simulink subsystem "F16_Quaternion"  (R2023b)
settings: Solver=VariableStepAuto  StartTime=0.0  StopTime=10.0  RelTol=1e-3
undefined symbols (not defined in the file): controlDeflections, dataBase, deltaLEF, e0_0, e1_0, e2_0, e3_0, pm_0, statesFinal, Vm_0, xme_0
libraries: sharedtransform x4, aerolibtransform2 x2, matrix_library x2, shared6dof x1
(part 2 of 2)

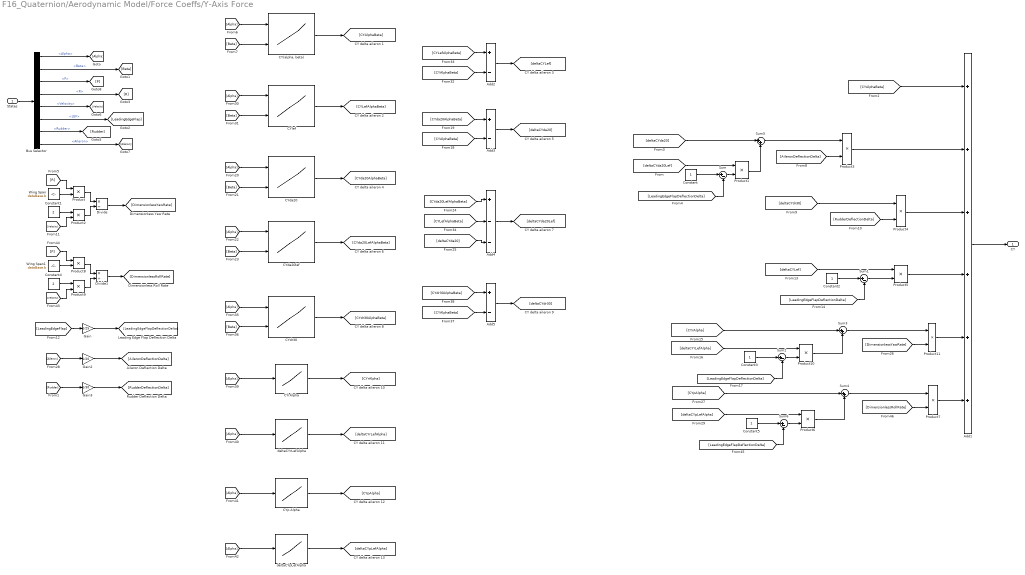
== system F16_Quaternion/Aerodynamic Model/Force Coeffs/Y-Axis Force ==
  States : Inport
  Add1 : Sum  Inputs=++++++
  Add2 : Sum  Inputs=+-
  Add3 : Sum  Inputs=+-
  Add4 : Sum  Inputs=+--
  Add5 : Sum  Inputs=+-
  Bus Selector : BusSelector  OutputSignals=Alpha,Beta,P,R,Velocity,LEF,Rudder,Aileron
  "CY(alpha, beta)" : Lookup_n-D  BreakpointsForDimension1=dataBase.f16_AerodynamicData.BP.CY.CY.alpha  BreakpointsForDimension2=dataBase.f16_AerodynamicData.BP.CY.CY.beta  Table=dataBase.f16_AerodynamicData.data.CY.CY  InternalRulePriority=Speed  RndMeth=Simplest
      settings: InputPortMap=u0,u1
  CYda20 : Lookup_n-D  BreakpointsForDimension1=dataBase.f16_AerodynamicData.BP.CY.CYda20.alpha  BreakpointsForDimension2=dataBase.f16_AerodynamicData.BP.CY.CYda20.beta  Table=dataBase.f16_AerodynamicData.data.CY.CYda20  InternalRulePriority=Speed  RndMeth=Simplest
      settings: InputPortMap=u0,u1
  CYda20lef : Lookup_n-D  BreakpointsForDimension1=dataBase.f16_AerodynamicData.BP.CY.CYda20lef.alpha  BreakpointsForDimension2=dataBase.f16_AerodynamicData.BP.CY.CYda20lef.beta  Table=dataBase.f16_AerodynamicData.data.CY.CYda20lef  InternalRulePriority=Speed  RndMeth=Simplest
      settings: InputPortMap=u0,u1
  CYdr30 : Lookup_n-D  BreakpointsForDimension1=dataBase.f16_AerodynamicData.BP.CY.CYdr30.alpha  BreakpointsForDimension2=dataBase.f16_AerodynamicData.BP.CY.CYdr30.beta  Table=dataBase.f16_AerodynamicData.data.CY.CYdr30  InternalRulePriority=Speed  RndMeth=Simplest
      settings: InputPortMap=u0,u1
  CYlef : Lookup_n-D  BreakpointsForDimension1=dataBase.f16_AerodynamicData.BP.CY.CYlef.alpha  BreakpointsForDimension2=dataBase.f16_AerodynamicData.BP.CY.CYlef.beta  Table=dataBase.f16_AerodynamicData.data.CY.CYlef  InternalRulePriority=Speed  RndMeth=Simplest
      settings: InputPortMap=u0,u1
  CYp Alpha : Lookup_n-D  NumberOfTableDimensions=1  BreakpointsForDimension1=dataBase.f16_AerodynamicData.BP.CY.CYp.alpha  Table=dataBase.f16_AerodynamicData.data.CY.CYp  InternalRulePriority=Speed  RndMeth=Simplest
  CYrAlpha : Lookup_n-D  NumberOfTableDimensions=1  BreakpointsForDimension1=dataBase.f16_AerodynamicData.BP.CY.CYr.alpha  Table=dataBase.f16_AerodynamicData.data.CY.CYr  InternalRulePriority=Speed  RndMeth=Simplest
  Constant{,2..3,5} (4 alike) : Constant
  Constant1 : Constant  Value=2
  Constant4 : Constant  Value=2
  Divide : Product  Inputs=*/
  Divide1 : Product  Inputs=*/
  Gain : Gain  Gain=1/25
  Gain2 : Gain  Gain=1/20
  Gain3 : Gain  Gain=1/30
  Product{,1..11} (12 alike) : Product
  Sum{,1..2,6} (4 alike) : Sum  Inputs=|+-
  Sum3 : Sum  Inputs=|++
  Sum4 : Sum  Inputs=|++
  Sum5 : Sum  Inputs=|++
  Wing Span : Constant  Value=dataBase.b
  Wing Span1 : Constant  Value=dataBase.b
  deltaCYpLefAlpha : Lookup_n-D  NumberOfTableDimensions=1  BreakpointsForDimension1=dataBase.f16_AerodynamicData.BP.CY.deltaCYplef.alpha  Table=dataBase.f16_AerodynamicData.data.CY.deltaCYplef  InternalRulePriority=Speed  RndMeth=Simplest
  deltaCYrLefAlpha : Lookup_n-D  NumberOfTableDimensions=1  BreakpointsForDimension1=dataBase.f16_AerodynamicData.BP.CY.deltaCYrlef.alpha  Table=dataBase.f16_AerodynamicData.data.CY.deltaCYrlef  InternalRulePriority=Speed  RndMeth=Simplest
  CY : Outport  VectorParamsAs1DForOutWhenUnconnected=off
  wires:
  Wing Span/1 -> Product/2
  Divide/1 -> [DimensionlessYawRate]
  [LeadingEdgeFlap] -> Gain/1
  Constant1/1 -> Product2/1
  [Beta] -> "CY(alpha, beta)"/2
  [R] -> Product/1
  States/1 -> Bus Selector/1
  Product2/1 -> Divide/2
  Product/1 -> Divide/1
  [Alpha] -> "CY(alpha, beta)"/1
  Gain/1 -> [LeadingEdgeFlapDeflectionDelta]
  [Velocity] -> Product2/2
  Add1/1 -> CY/1
  "CY(alpha, beta)"/1 -> [CYAlphaBeta]
  [Beta] -> CYda20/2
  [Alpha] -> CYda20/1
  [Alpha] -> CYda20lef/1
  [Beta] -> CYda20lef/2
  [Aileron] -> Gain2/1
  Gain2/1 -> [AileronDeflectionDelta]
  [Alpha] -> CYlef/1
  [Beta] -> CYlef/2
  CYlef/1 -> [CYLefAlphaBeta]
  Add2/1 -> [deltaCYLef]
  [CYAlphaBeta] -> Add2/2
  [CYLefAlphaBeta] -> Add2/1
  CYda20/1 -> [CYda20AlphaBeta]
  [CYda20AlphaBeta] -> Add3/1
  [CYAlphaBeta] -> Add3/2
  Add3/1 -> [deltaCYda20]
  CYda20lef/1 -> [CYda20LefAlphaBeta]
  [CYda20LefAlphaBeta] -> Add4/1
  [CYLefAlphaBeta] -> Add4/2
  [deltaCYda20] -> Add4/3
  Add4/1 -> [deltaCYda20Lef]
  CYdr30/1 -> [CYdr30AlphaBeta]
  [Alpha] -> CYdr30/1
  [Beta] -> CYdr30/2
  Add5/1 -> [deltaCYdr30]
  [CYAlphaBeta] -> Add5/2
  [CYdr30AlphaBeta] -> Add5/1
  [Alpha] -> CYrAlpha/1
  CYrAlpha/1 -> [CYrAlpha]
  deltaCYrLefAlpha/1 -> [deltaCYrLefAlpha]
  [Alpha] -> deltaCYrLefAlpha/1
  [Alpha] -> deltaCYpLefAlpha/1
  deltaCYpLefAlpha/1 -> [deltaCYpLefAlpha]
  CYp Alpha/1 -> [CYpAlpha]
  [Alpha] -> CYp Alpha/1
  [Velocity] -> Product9/2
  Product8/1 -> Divide1/1
  Product9/1 -> Divide1/2
  [P] -> Product8/1
  Constant4/1 -> Product9/1
  Divide1/1 -> [DimensionlessRollRate]
  Wing Span1/1 -> Product8/2
  Gain3/1 -> [RudderDeflectionDelta]
  [Rudder] -> Gain3/1
  [CYAlphaBeta] -> Add1/1
  [deltaCYda20Lef] -> Product1/1
  [deltaCYda20] -> Sum5/1
  Product1/1 -> Sum5/2
  Sum5/1 -> Product3/1
  [AileronDeflectionDelta] -> Product3/2
  Product3/1 -> Add1/2
  [RudderDeflectionDelta] -> Product4/2
  [deltaCYdr30] -> Product4/1
  Product4/1 -> Add1/3
  [deltaCYLef] -> Product5/1
  Product5/1 -> Add1/4
  [CYrAlpha] -> Sum3/1
  [deltaCYrLefAlpha] -> Product10/1
  Product10/1 -> Sum3/2
  [DimensionlessYawRate] -> Product11/2
  Sum3/1 -> Product11/1
  Product11/1 -> Add1/5
  Product7/1 -> Add1/6
  Sum4/1 -> Product7/1
  [DimensionlessRollRate] -> Product7/2
  Product6/1 -> Sum4/2
  [deltaCYpLefAlpha] -> Product6/1
  [CYpAlpha] -> Sum4/1
  Constant/1 -> Sum/1
  [LeadingEdgeFlapDeflectionDelta] -> Sum/2
  Sum/1 -> Product1/2
  Constant2/1 -> Sum1/1
  [LeadingEdgeFlapDeflectionDelta] -> Sum1/2
  Sum1/1 -> Product5/2
  Constant3/1 -> Sum2/1
  [LeadingEdgeFlapDeflectionDelta] -> Sum2/2
  Sum2/1 -> Product10/2
  Constant5/1 -> Sum6/1
  [LeadingEdgeFlapDeflectionDelta] -> Sum6/2
  Sum6/1 -> Product6/2
  Bus Selector/1 -> [Alpha]  "<Alpha>"
  Bus Selector/2 -> [Beta]  "<Beta>"
  Bus Selector/3 -> [P]  "<P>"
  Bus Selector/4 -> [R]  "<R>"
  Bus Selector/5 -> [Velocity]  "<Velocity>"
  Bus Selector/6 -> [LeadingEdgeFlap]  "<LEF>"
  Bus Selector/7 -> [Rudder]  "<Rudder>"
  Bus Selector/8 -> [Aileron]  "<Aileron>"

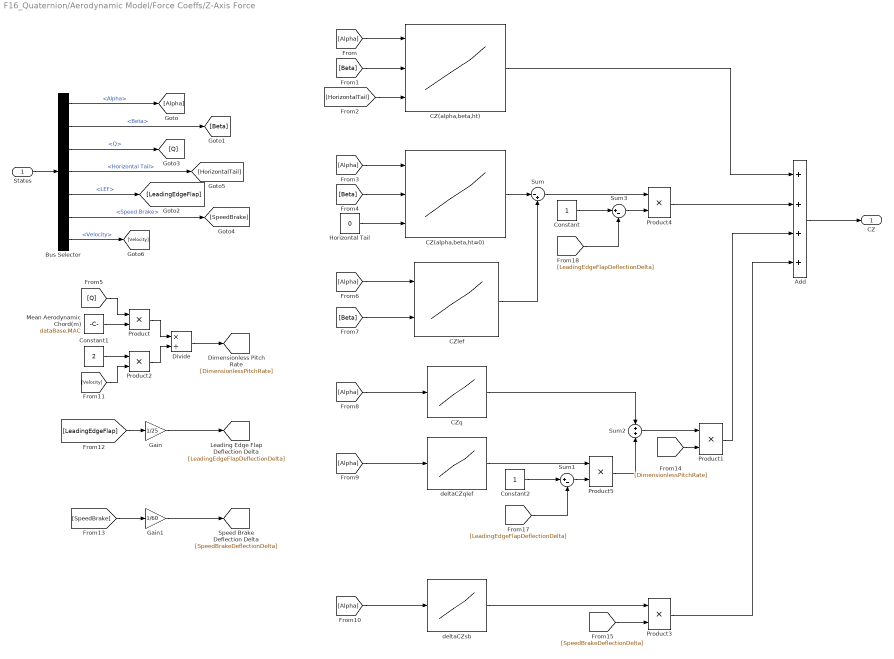
== system F16_Quaternion/Aerodynamic Model/Force Coeffs/Z-Axis Force ==
  States : Inport
  Add : Sum  Inputs=++++
  Bus Selector : BusSelector  OutputSignals=Alpha,Beta,Q,Horizontal Tail,LEF,Speed Brake,Velocity
  CZ(alpha,beta,ht) : Lookup_n-D  NumberOfTableDimensions=3  BreakpointsForDimension1=dataBase.f16_AerodynamicData.BP.CZ.CZ.alpha  BreakpointsForDimension2=dataBase.f16_AerodynamicData.BP.CZ.CZ.beta  BreakpointsForDimension3=dataBase.f16_AerodynamicData.BP.CZ.CZ.dHT  Table=dataBase.f16_AerodynamicData.data.CZ.CZ  InternalRulePriority=Speed  RndMeth=Simplest
      settings: InputPortMap=u0,u1,u2
  CZ(alpha,beta,ht=0) : Lookup_n-D  NumberOfTableDimensions=3  BreakpointsForDimension1=dataBase.f16_AerodynamicData.BP.CZ.CZ.alpha  BreakpointsForDimension2=dataBase.f16_AerodynamicData.BP.CZ.CZ.beta  BreakpointsForDimension3=dataBase.f16_AerodynamicData.BP.CZ.CZ.dHT  Table=dataBase.f16_AerodynamicData.data.CZ.CZ  InternalRulePriority=Speed  RndMeth=Simplest
      settings: InputPortMap=u0,u1,u2
  CZlef : Lookup_n-D  BreakpointsForDimension1=dataBase.f16_AerodynamicData.BP.CZ.CZlef.alpha  BreakpointsForDimension2=dataBase.f16_AerodynamicData.BP.CZ.CZlef.beta  Table=dataBase.f16_AerodynamicData.data.CZ.CZlef  InternalRulePriority=Speed  RndMeth=Simplest
      settings: InputPortMap=u0,u1
  CZq : Lookup_n-D  NumberOfTableDimensions=1  BreakpointsForDimension1=dataBase.f16_AerodynamicData.BP.CZ.CZq.alpha  Table=dataBase.f16_AerodynamicData.data.CZ.CZq  InternalRulePriority=Speed  RndMeth=Simplest
  Constant : Constant
  Constant1 : Constant  Value=2
  Constant2 : Constant
  Divide : Product  Inputs=*/
  Gain : Gain  Gain=1/25
  Gain1 : Gain  Gain=1/60
  Horizontal Tail : Constant  Value=0
  Mean Aerodynamic Chord(m) : Constant  Value=dataBase.MAC
  Product{,1..5} (6 alike) : Product
  Sum : Sum  Inputs=|-+
  Sum1 : Sum  Inputs=|+-
  Sum2 : Sum  Inputs=+|+
  Sum3 : Sum  Inputs=|+-
  deltaCZqlef : Lookup_n-D  NumberOfTableDimensions=1  BreakpointsForDimension1=dataBase.f16_AerodynamicData.BP.CZ.deltaCZqlef.alpha  Table=dataBase.f16_AerodynamicData.data.CZ.deltaCZqlef  InternalRulePriority=Speed  RndMeth=Simplest
  deltaCZsb : Lookup_n-D  NumberOfTableDimensions=1  BreakpointsForDimension1=dataBase.f16_AerodynamicData.BP.CZ.deltaCZSB.alpha  Table=dataBase.f16_AerodynamicData.data.CZ.deltaCZSB  InternalRulePriority=Speed  RndMeth=Simplest
  CZ : Outport  VectorParamsAs1DForOutWhenUnconnected=off
  wires:
  [Beta] -> CZ(alpha,beta,ht=0)/2
  Product2/1 -> Divide/2
  [Alpha] -> CZlef/1
  [Velocity] -> Product2/2
  Sum2/1 -> Product1/1
  [SpeedBrake] -> Gain1/1
  Product/1 -> Divide/1
  [LeadingEdgeFlap] -> Gain/1
  Divide/1 -> [DimensionlessPitchRate]
  Mean Aerodynamic Chord(m)/1 -> Product/2
  [Alpha] -> deltaCZsb/1
  [HorizontalTail] -> CZ(alpha,beta,ht)/3
  CZlef/1 -> Sum/2
  Constant1/1 -> Product2/1
  [Beta] -> CZ(alpha,beta,ht)/2
  Horizontal Tail/1 -> CZ(alpha,beta,ht=0)/3
  [Alpha] -> CZ(alpha,beta,ht=0)/1
  [Alpha] -> CZq/1
  [Alpha] -> deltaCZqlef/1
  [Alpha] -> CZ(alpha,beta,ht)/1
  States/1 -> Bus Selector/1
  CZ(alpha,beta,ht=0)/1 -> Sum/1
  Sum/1 -> Product4/1
  Product3/1 -> Add/4
  CZq/1 -> Sum2/1
  Gain1/1 -> [SpeedBrakeDeflectionDelta]
  CZ(alpha,beta,ht)/1 -> Add/1
  Add/1 -> CZ/1
  deltaCZsb/1 -> Product3/1
  [SpeedBrakeDeflectionDelta] -> Product3/2
  [Q] -> Product/1
  [DimensionlessPitchRate] -> Product1/2
  [Beta] -> CZlef/2
  Product1/1 -> Add/3
  Gain/1 -> [LeadingEdgeFlapDeflectionDelta]
  Product4/1 -> Add/2
  deltaCZqlef/1 -> Product5/1
  Product5/1 -> Sum2/2
  Sum3/1 -> Product4/2
  [LeadingEdgeFlapDeflectionDelta] -> Sum3/2
  Constant/1 -> Sum3/1
  Sum1/1 -> Product5/2
  [LeadingEdgeFlapDeflectionDelta] -> Sum1/2
  Constant2/1 -> Sum1/1
  Bus Selector/1 -> [Alpha]  "<Alpha>"
  Bus Selector/2 -> [Beta]  "<Beta>"
  Bus Selector/3 -> [Q]  "<Q>"
  Bus Selector/4 -> [HorizontalTail]  "<Horizontal Tail>"
  Bus Selector/5 -> [LeadingEdgeFlap]  "<LEF>"
  Bus Selector/7 -> [Velocity]  "<Velocity>"
  Bus Selector/6 -> [SpeedBrake]  "<Speed Brake>"

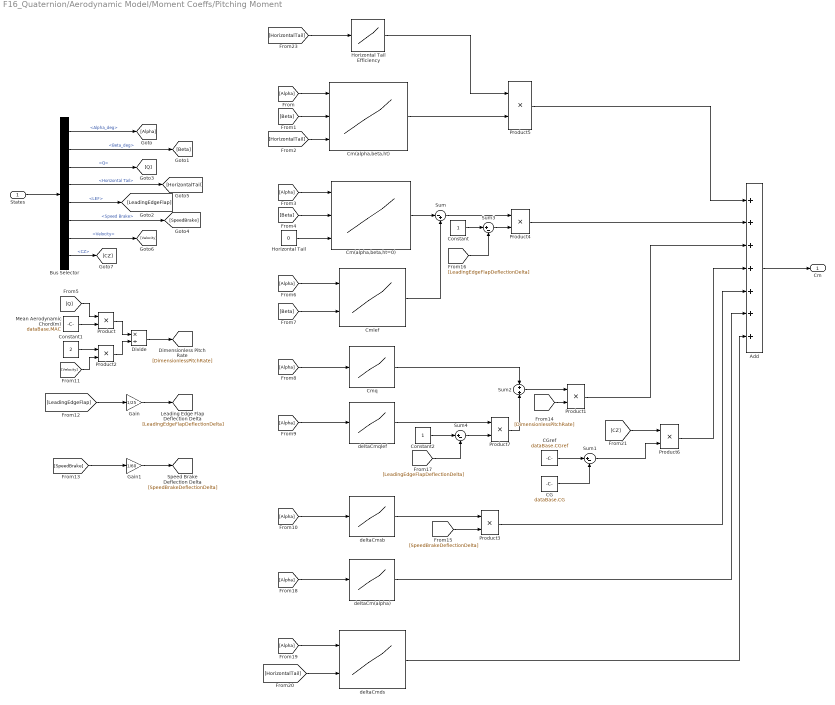
== system F16_Quaternion/Aerodynamic Model/Moment Coeffs/Pitching Moment ==
  States : Inport
  Add : Sum  Inputs=+++++++
  Bus Selector : BusSelector  OutputSignals=Alpha_deg,Beta_deg,Q,Horizontal Tail,LEF,Speed Brake,Velocity,CZ
  CG : Constant  Value=dataBase.CG
  CGref : Constant  Value=dataBase.CGref
  Cm(alpha,beta,ht) : Lookup_n-D  NumberOfTableDimensions=3  BreakpointsForDimension1=dataBase.f16_AerodynamicData.BP.Cm.Cm.alpha  BreakpointsForDimension2=dataBase.f16_AerodynamicData.BP.Cm.Cm.beta  BreakpointsForDimension3=dataBase.f16_AerodynamicData.BP.Cm.Cm.dHT  Table=dataBase.f16_AerodynamicData.data.Cm.Cm  ExtrapMethod=Clip  InternalRulePriority=Speed  RndMeth=Simplest
      settings: InputPortMap=u0,u1,u2
  Cm(alpha,beta,ht=0) : Lookup_n-D  NumberOfTableDimensions=3  BreakpointsForDimension1=dataBase.f16_AerodynamicData.BP.Cm.Cm.alpha  BreakpointsForDimension2=dataBase.f16_AerodynamicData.BP.Cm.Cm.beta  BreakpointsForDimension3=dataBase.f16_AerodynamicData.BP.Cm.Cm.dHT  Table=dataBase.f16_AerodynamicData.data.Cm.Cm  ExtrapMethod=Clip  InternalRulePriority=Speed  RndMeth=Simplest
      settings: InputPortMap=u0,u1,u2
  Cmlef : Lookup_n-D  BreakpointsForDimension1=dataBase.f16_AerodynamicData.BP.Cm.Cmlef.alpha  BreakpointsForDimension2=dataBase.f16_AerodynamicData.BP.Cm.Cmlef.beta  Table=dataBase.f16_AerodynamicData.data.Cm.Cmlef  ExtrapMethod=Clip  InternalRulePriority=Speed  RndMeth=Simplest
      settings: InputPortMap=u0,u1
  Cmq : Lookup_n-D  NumberOfTableDimensions=1  BreakpointsForDimension1=dataBase.f16_AerodynamicData.BP.Cm.Cmq.alpha  Table=dataBase.f16_AerodynamicData.data.Cm.Cmq  ExtrapMethod=Clip  InternalRulePriority=Speed  RndMeth=Simplest
  Constant : Constant
  Constant1 : Constant  Value=2
  Constant2 : Constant
  Divide : Product  Inputs=*/
  Gain : Gain  Gain=1/25
  Gain1 : Gain  Gain=1/60
  Horizontal Tail : Constant  Value=0
  Horizontal Tail Efficiency : Lookup_n-D  NumberOfTableDimensions=1  BreakpointsForDimension1=dataBase.f16_AerodynamicData.BP.Cm.n_dHT.dHT  Table=dataBase.f16_AerodynamicData.data.Cm.n_dHT  ExtrapMethod=Clip  InternalRulePriority=Speed  RndMeth=Simplest
  Mean Aerodynamic Chord(m) : Constant  Value=dataBase.MAC
  Product{,1..7} (8 alike) : Product
  Sum : Sum  Inputs=|-+
  Sum1 : Sum  Inputs=|+-
  Sum2 : Sum  Inputs=+|+
  Sum3 : Sum  Inputs=|+-
  Sum4 : Sum  Inputs=|+-
  deltaCm(alpha) : Lookup_n-D  NumberOfTableDimensions=1  BreakpointsForDimension1=dataBase.f16_AerodynamicData.BP.Cm.deltaCm.alpha  Table=dataBase.f16_AerodynamicData.data.Cm.deltaCm  ExtrapMethod=Clip  InternalRulePriority=Speed  RndMeth=Simplest
  deltaCmds : Lookup_n-D  BreakpointsForDimension1=dataBase.f16_AerodynamicData.BP.Cm.deltaCmds.alpha  BreakpointsForDimension2=dataBase.f16_AerodynamicData.BP.Cm.deltaCmds.dHT  Table=dataBase.f16_AerodynamicData.data.Cm.deltaCmds  ExtrapMethod=Clip  InternalRulePriority=Speed  RndMeth=Simplest
      settings: InputPortMap=u0,u1
  deltaCmqlef : Lookup_n-D  NumberOfTableDimensions=1  BreakpointsForDimension1=dataBase.f16_AerodynamicData.BP.Cm.deltaCmqlef.alpha  Table=dataBase.f16_AerodynamicData.data.Cm.deltaCmqlef  ExtrapMethod=Clip  InternalRulePriority=Speed  RndMeth=Simplest
  deltaCmsb : Lookup_n-D  NumberOfTableDimensions=1  BreakpointsForDimension1=dataBase.f16_AerodynamicData.BP.Cm.deltaCmSB.alpha  Table=dataBase.f16_AerodynamicData.data.Cm.deltaCmSB  ExtrapMethod=Clip  InternalRulePriority=Speed  RndMeth=Simplest
  Cm : Outport
  wires:
  [Beta] -> Cm(alpha,beta,ht=0)/2
  [SpeedBrakeDeflectionDelta] -> Product3/2
  Constant1/1 -> Product2/1
  [Alpha] -> Cm(alpha,beta,ht=0)/1
  Product/1 -> Divide/1
  Cm(alpha,beta,ht=0)/1 -> Sum/1
  Horizontal Tail/1 -> Cm(alpha,beta,ht=0)/3
  [Alpha] -> Cm(alpha,beta,ht)/1
  States/1 -> Bus Selector/1
  [Alpha] -> Cmlef/1
  [Alpha] -> deltaCmqlef/1
  [Alpha] -> Cmq/1
  Mean Aerodynamic Chord(m)/1 -> Product/2
  Product1/1 -> Add/3
  Sum2/1 -> Product1/1
  [Q] -> Product/1
  Gain1/1 -> [SpeedBrakeDeflectionDelta]
  Cmlef/1 -> Sum/2
  [DimensionlessPitchRate] -> Product1/2
  [Beta] -> Cm(alpha,beta,ht)/2
  Divide/1 -> [DimensionlessPitchRate]
  Product4/1 -> Add/2
  Add/1 -> Cm/1
  [LeadingEdgeFlap] -> Gain/1
  [HorizontalTail] -> Cm(alpha,beta,ht)/3
  [SpeedBrake] -> Gain1/1
  Product2/1 -> Divide/2
  Gain/1 -> [LeadingEdgeFlapDeflectionDelta]
  [Velocity] -> Product2/2
  deltaCmsb/1 -> Product3/1
  Sum/1 -> Product4/1
  [Alpha] -> deltaCmsb/1
  Cmq/1 -> Sum2/1
  [Beta] -> Cmlef/2
  [Alpha] -> deltaCm(alpha)/1
  [HorizontalTail] -> deltaCmds/2
  [Alpha] -> deltaCmds/1
  Product5/1 -> Add/1
  [CZ] -> Product6/1
  CGref/1 -> Sum1/1
  CG/1 -> Sum1/2
  deltaCmqlef/1 -> Product7/1
  Product7/1 -> Sum2/2
  [HorizontalTail] -> Horizontal Tail Efficiency/1
  Cm(alpha,beta,ht)/1 -> Product5/2
  Horizontal Tail Efficiency/1 -> Product5/1
  Constant/1 -> Sum3/1
  [LeadingEdgeFlapDeflectionDelta] -> Sum3/2
  Sum3/1 -> Product4/2
  Constant2/1 -> Sum4/1
  Sum4/1 -> Product7/2
  [LeadingEdgeFlapDeflectionDelta] -> Sum4/2
  Product6/1 -> Add/4
  Product3/1 -> Add/5
  deltaCm(alpha)/1 -> Add/6
  deltaCmds/1 -> Add/7
  Bus Selector/1 -> [Alpha]  "<Alpha_deg>"
  Bus Selector/2 -> [Beta]  "<Beta_deg>"
  Bus Selector/3 -> [Q]  "<Q>"
  Bus Selector/4 -> [HorizontalTail]  "<Horizontal Tail>"
  Bus Selector/5 -> [LeadingEdgeFlap]  "<LEF>"
  Bus Selector/6 -> [SpeedBrake]  "<Speed Brake>"
  Bus Selector/7 -> [Velocity]  "<Velocity>"
  Bus Selector/8 -> [CZ]  "<CZ>"
  Sum1/1 -> Product6/2

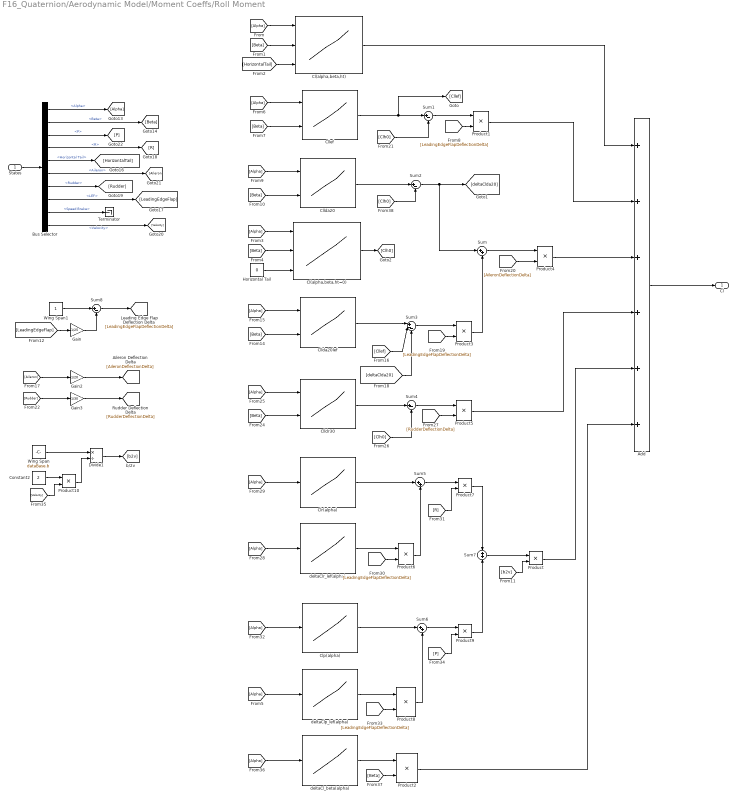
== system F16_Quaternion/Aerodynamic Model/Moment Coeffs/Roll Moment ==
  States : Inport
  Add : Sum  Inputs=++++++
  Bus Selector : BusSelector  OutputSignals=Alpha,Beta,P,R,Horizontal Tail,Aileron,Rudder,LEF,Speed Brake,Velocity
  Cl(alpha,beta,ht) : Lookup_n-D  NumberOfTableDimensions=3  BreakpointsForDimension1=dataBase.f16_AerodynamicData.BP.Cl.Cl.alpha  BreakpointsForDimension2=dataBase.f16_AerodynamicData.BP.Cl.Cl.beta  BreakpointsForDimension3=dataBase.f16_AerodynamicData.BP.Cl.Cl.dHT  Table=dataBase.f16_AerodynamicData.data.Cl.Cl  ExtrapMethod=Clip  InternalRulePriority=Speed  RndMeth=Simplest
      settings: InputPortMap=u0,u1,u2
  Cl(alpha,beta,ht=0) : Lookup_n-D  NumberOfTableDimensions=3  BreakpointsForDimension1=dataBase.f16_AerodynamicData.BP.Cl.Cl.alpha  BreakpointsForDimension2=dataBase.f16_AerodynamicData.BP.Cl.Cl.beta  BreakpointsForDimension3=dataBase.f16_AerodynamicData.BP.Cl.Cl.dHT  Table=dataBase.f16_AerodynamicData.data.Cl.Cl  ExtrapMethod=Clip  InternalRulePriority=Speed  RndMeth=Simplest
      settings: InputPortMap=u0,u1,u2
  Cllda20 : Lookup_n-D  BreakpointsForDimension1=dataBase.f16_AerodynamicData.BP.Cl.Clda20.alpha  BreakpointsForDimension2=dataBase.f16_AerodynamicData.BP.Cl.Clda20.beta  Table=dataBase.f16_AerodynamicData.data.Cl.Clda20  ExtrapMethod=Clip  InternalRulePriority=Speed  RndMeth=Simplest
      settings: InputPortMap=u0,u1
  Cllda20lef : Lookup_n-D  BreakpointsForDimension1=dataBase.f16_AerodynamicData.BP.Cl.Clda20lef.alpha  BreakpointsForDimension2=dataBase.f16_AerodynamicData.BP.Cl.Clda20lef.beta  Table=dataBase.f16_AerodynamicData.data.Cl.Clda20lef  ExtrapMethod=Clip  InternalRulePriority=Speed  RndMeth=Simplest
      settings: InputPortMap=u0,u1
  Clldr30 : Lookup_n-D  BreakpointsForDimension1=dataBase.f16_AerodynamicData.BP.Cl.Cldr30.alpha  BreakpointsForDimension2=dataBase.f16_AerodynamicData.BP.Cl.Cldr30.beta  Table=dataBase.f16_AerodynamicData.data.Cl.Cldr30  ExtrapMethod=Clip  InternalRulePriority=Speed  RndMeth=Simplest
      settings: InputPortMap=u0,u1
  Cllef : Lookup_n-D  BreakpointsForDimension1=dataBase.f16_AerodynamicData.BP.Cl.Cllef.alpha  BreakpointsForDimension2=dataBase.f16_AerodynamicData.BP.Cl.Cllef.beta  Table=dataBase.f16_AerodynamicData.data.Cl.Cllef  ExtrapMethod=Clip  InternalRulePriority=Speed  RndMeth=Simplest
      settings: InputPortMap=u0,u1
  Clp(alpha) : Lookup_n-D  NumberOfTableDimensions=1  BreakpointsForDimension1=dataBase.f16_AerodynamicData.BP.Cl.Clp.alpha  BreakpointsForDimension2=dataBase.f16_AerodynamicData.BP.Cl.Cldr30.beta  Table=dataBase.f16_AerodynamicData.data.Cl.Clp  ExtrapMethod=Clip  InternalRulePriority=Speed  RndMeth=Simplest
  Clr(alpha) : Lookup_n-D  NumberOfTableDimensions=1  BreakpointsForDimension1=dataBase.f16_AerodynamicData.BP.Cl.Clr.alpha  BreakpointsForDimension2=dataBase.f16_AerodynamicData.BP.Cl.Cldr30.beta  Table=dataBase.f16_AerodynamicData.data.Cl.Clr  ExtrapMethod=Clip  InternalRulePriority=Speed  RndMeth=Simplest
  Constant2 : Constant  Value=2
  Divide1 : Product  Inputs=*/
  Gain : Gain  Gain=1/25
  Gain2 : Gain  Gain=1/20
  Gain3 : Gain  Gain=1/30
  Horizontal Tail : Constant  Value=0
  Product{,1..10} (11 alike) : Product
  Sum : Sum  Inputs=|++
  Sum{1..2,4,8} (4 alike) : Sum  Inputs=|+-
  Sum3 : Sum  Inputs=|+--
  Sum5 : Sum  Inputs=|++
  Sum6 : Sum  Inputs=|++
  Sum7 : Sum  Inputs=+|+
  Terminator : Terminator
  Wing Span : Constant  Value=dataBase.b
  Wing Span1 : Constant
  deltaCl_beta(alpha) : Lookup_n-D  NumberOfTableDimensions=1  BreakpointsForDimension1=dataBase.f16_AerodynamicData.BP.Cl.deltaClBeta.alpha  BreakpointsForDimension2=dataBase.f16_AerodynamicData.BP.Cl.Cldr30.beta  Table=dataBase.f16_AerodynamicData.data.Cl.deltaClBeta  ExtrapMethod=Clip  InternalRulePriority=Speed  RndMeth=Simplest
  deltaClp_lef(alpha) : Lookup_n-D  NumberOfTableDimensions=1  BreakpointsForDimension1=dataBase.f16_AerodynamicData.BP.Cl.deltaClplef.alpha  BreakpointsForDimension2=dataBase.f16_AerodynamicData.BP.Cl.Cldr30.beta  Table=dataBase.f16_AerodynamicData.data.Cl.deltaClplef  ExtrapMethod=Clip  InternalRulePriority=Speed  RndMeth=Simplest
  deltaClr_lef(alpha) : Lookup_n-D  NumberOfTableDimensions=1  BreakpointsForDimension1=dataBase.f16_AerodynamicData.BP.Cl.deltaClrlef.alpha  BreakpointsForDimension2=dataBase.f16_AerodynamicData.BP.Cl.Cldr30.beta  Table=dataBase.f16_AerodynamicData.data.Cl.deltaClrlef  ExtrapMethod=Clip  InternalRulePriority=Speed  RndMeth=Simplest
  Cl : Outport
  wires:
  [Beta] -> Cllef/2
  [HorizontalTail] -> Cl(alpha,beta,ht)/3
  Cl(alpha,beta,ht)/1 -> Add/1
  [Alpha] -> Cllef/1
  [Alpha] -> Cl(alpha,beta,ht)/1
  [Beta] -> Cl(alpha,beta,ht)/2
  Add/1 -> Cl/1
  Gain/1 -> Sum8/2
  [LeadingEdgeFlap] -> Gain/1
  [Aileron] -> Gain2/1
  Gain2/1 -> [AileronDeflectionDelta]
  Gain3/1 -> [RudderDeflectionDelta]
  [Rudder] -> Gain3/1
  [Beta] -> Cl(alpha,beta,ht=0)/2
  Horizontal Tail/1 -> Cl(alpha,beta,ht=0)/3
  [Alpha] -> Cl(alpha,beta,ht=0)/1
  Cllef/1 -> Sum1/1, [Cllef]
  [LeadingEdgeFlapDeflectionDelta] -> Product1/2
  Sum1/1 -> Product1/1
  Cl(alpha,beta,ht=0)/1 -> [Clh0]
  [Beta] -> Cllda20/2
  [Alpha] -> Cllda20/1
  Cllda20/1 -> Sum2/1
  Product1/1 -> Add/2
  Sum2/1 -> Sum/1, [deltaClda20]
  [Alpha] -> Cllda20lef/1
  [Beta] -> Cllda20lef/2
  Cllda20lef/1 -> Sum3/1
  [Cllef] -> Sum3/2
  [deltaClda20] -> Sum3/3
  [LeadingEdgeFlapDeflectionDelta] -> Product3/2
  Sum3/1 -> Product3/1
  Product3/1 -> Sum/2
  [AileronDeflectionDelta] -> Product4/2
  Sum/1 -> Product4/1
  Product4/1 -> Add/3
  [Clh0] -> Sum1/2
  [Clh0] -> Sum2/2
  [Alpha] -> Clldr30/1
  [Beta] -> Clldr30/2
  Clldr30/1 -> Sum4/1
  [Clh0] -> Sum4/2
  [RudderDeflectionDelta] -> Product5/2
  Sum4/1 -> Product5/1
  Product5/1 -> Add/4
  [Alpha] -> Clr(alpha)/1
  Clr(alpha)/1 -> Sum5/1
  [Alpha] -> deltaClr_lef(alpha)/1
  [LeadingEdgeFlapDeflectionDelta] -> Product6/2
  deltaClr_lef(alpha)/1 -> Product6/1
  Product6/1 -> Sum5/2
  [Alpha] -> Clp(alpha)/1
  [Alpha] -> deltaClp_lef(alpha)/1
  [LeadingEdgeFlapDeflectionDelta] -> Product8/2
  deltaClp_lef(alpha)/1 -> Product8/1
  Product8/1 -> Sum6/2
  Clp(alpha)/1 -> Sum6/1
  Sum6/1 -> Product9/1
  [P] -> Product9/2
  Sum5/1 -> Product7/1
  [R] -> Product7/2
  Product7/1 -> Sum7/1
  Product9/1 -> Sum7/2
  [Velocity] -> Product10/2
  Constant2/1 -> Product10/1
  Product10/1 -> Divide1/2
  Wing Span/1 -> Divide1/1
  Divide1/1 -> [b2v]
  Sum7/1 -> Product/1
  [b2v] -> Product/2
  [Alpha] -> deltaCl_beta(alpha)/1
  deltaCl_beta(alpha)/1 -> Product2/1
  [Beta] -> Product2/2
  Product/1 -> Add/5
  Product2/1 -> Add/6
  Bus Selector/7 -> [Rudder]  "<Rudder>"
  Bus Selector/3 -> [P]  "<P>"
  Bus Selector/5 -> [HorizontalTail]  "<Horizontal Tail>"
  States/1 -> Bus Selector/1
  Bus Selector/2 -> [Beta]  "<Beta>"
  Bus Selector/10 -> [Velocity]  "<Velocity>"
  Bus Selector/1 -> [Alpha]  "<Alpha>"
  Bus Selector/6 -> [Aileron]  "<Aileron>"
  Bus Selector/8 -> [LeadingEdgeFlap]  "<LEF>"
  Bus Selector/4 -> [R]  "<R>"
  Bus Selector/9 -> Terminator/1  "<Speed Brake>"
  Wing Span1/1 -> Sum8/1
  Sum8/1 -> [LeadingEdgeFlapDeflectionDelta]

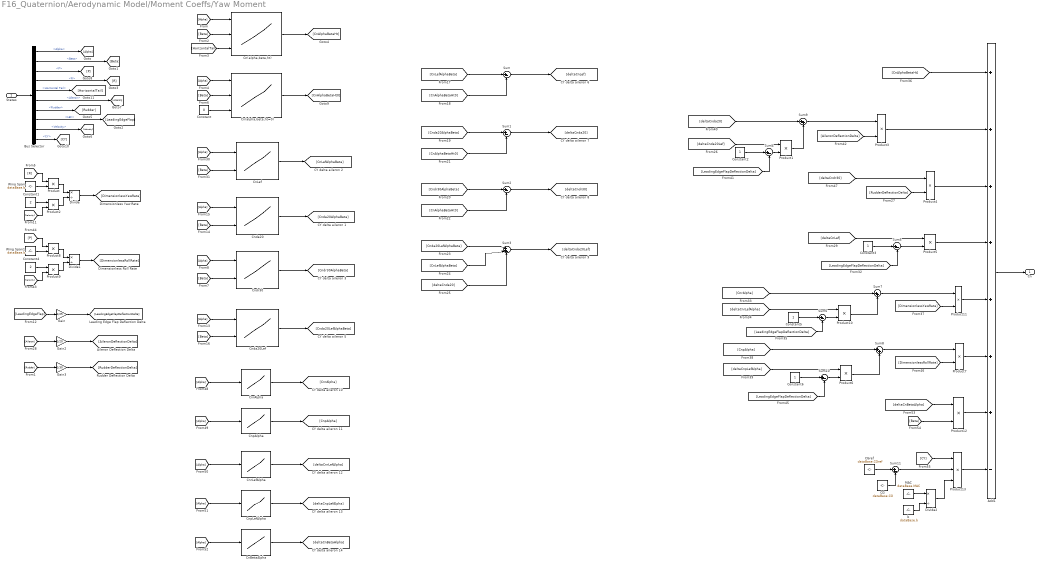
== system F16_Quaternion/Aerodynamic Model/Moment Coeffs/Yaw Moment ==
  States : Inport
  Add1 : Sum  Inputs=+++++++-
  Bus Selector : BusSelector  OutputSignals=Alpha,Beta,P,R,Horizontal Tail,Aileron,Rudder,LEF,Velocity,CY
  CG : Constant  Value=dataBase.CG
  CGref : Constant  Value=dataBase.CGref
  Cn(alpha,beta,ht) : Lookup_n-D  NumberOfTableDimensions=3  BreakpointsForDimension1=dataBase.f16_AerodynamicData.BP.Cn.Cn.alpha  BreakpointsForDimension2=dataBase.f16_AerodynamicData.BP.Cn.Cn.beta  BreakpointsForDimension3=dataBase.f16_AerodynamicData.BP.Cn.Cn.dHT  Table=dataBase.f16_AerodynamicData.data.Cn.Cn  ExtrapMethod=Clip  InternalRulePriority=Speed  RndMeth=Simplest
      settings: InputPortMap=u0,u1,u2
  Cn(alpha,beta,ht=0) : Lookup_n-D  NumberOfTableDimensions=3  BreakpointsForDimension1=dataBase.f16_AerodynamicData.BP.Cn.Cn.alpha  BreakpointsForDimension2=dataBase.f16_AerodynamicData.BP.Cn.Cn.beta  BreakpointsForDimension3=dataBase.f16_AerodynamicData.BP.Cn.Cn.dHT  Table=dataBase.f16_AerodynamicData.data.Cn.Cn  ExtrapMethod=Clip  InternalRulePriority=Speed  RndMeth=Simplest
      settings: InputPortMap=u0,u1,u2
  CnBetaAlpha : Lookup_n-D  NumberOfTableDimensions=1  BreakpointsForDimension1=dataBase.f16_AerodynamicData.BP.Cn.deltaCnBeta.alpha  Table=dataBase.f16_AerodynamicData.data.Cn.deltaCnBeta  ExtrapMethod=Clip  InternalRulePriority=Speed  RndMeth=Simplest
  CnLef : Lookup_n-D  BreakpointsForDimension1=dataBase.f16_AerodynamicData.BP.Cn.Cnlef.alpha  BreakpointsForDimension2=dataBase.f16_AerodynamicData.BP.Cn.Cnlef.beta  Table=dataBase.f16_AerodynamicData.data.Cn.Cnlef  ExtrapMethod=Clip  InternalRulePriority=Speed  RndMeth=Simplest
      settings: InputPortMap=u0,u1
  Cnda20 : Lookup_n-D  BreakpointsForDimension1=dataBase.f16_AerodynamicData.BP.Cn.Cnda20.alpha  BreakpointsForDimension2=dataBase.f16_AerodynamicData.BP.Cn.Cnda20.beta  Table=dataBase.f16_AerodynamicData.data.Cn.Cnda20  ExtrapMethod=Clip  InternalRulePriority=Speed  RndMeth=Simplest
      settings: InputPortMap=u0,u1
  Cnda20Lef : Lookup_n-D  BreakpointsForDimension1=dataBase.f16_AerodynamicData.BP.Cn.Cnda20lef.alpha  BreakpointsForDimension2=dataBase.f16_AerodynamicData.BP.Cn.Cnda20lef.beta  Table=dataBase.f16_AerodynamicData.data.Cn.Cnda20lef  ExtrapMethod=Clip  InternalRulePriority=Speed  RndMeth=Simplest
      settings: InputPortMap=u0,u1
  Cndr30 : Lookup_n-D  BreakpointsForDimension1=dataBase.f16_AerodynamicData.BP.Cn.Cndr30.alpha  BreakpointsForDimension2=dataBase.f16_AerodynamicData.BP.Cn.Cndr30.beta  Table=dataBase.f16_AerodynamicData.data.Cn.Cndr30  ExtrapMethod=Clip  InternalRulePriority=Speed  RndMeth=Simplest
      settings: InputPortMap=u0,u1
  CnpAlpha : Lookup_n-D  NumberOfTableDimensions=1  BreakpointsForDimension1=dataBase.f16_AerodynamicData.BP.Cn.Cnp.alpha  Table=dataBase.f16_AerodynamicData.data.Cn.Cnp  ExtrapMethod=Clip  InternalRulePriority=Speed  RndMeth=Simplest
  CnpLefAlpha : Lookup_n-D  NumberOfTableDimensions=1  BreakpointsForDimension1=dataBase.f16_AerodynamicData.BP.Cn.deltaCnplef.alpha  Table=dataBase.f16_AerodynamicData.data.Cn.deltaCnplef  ExtrapMethod=Clip  InternalRulePriority=Speed  RndMeth=Simplest
  CnrAlpha : Lookup_n-D  NumberOfTableDimensions=1  BreakpointsForDimension1=dataBase.f16_AerodynamicData.BP.Cn.Cnr.alpha  Table=dataBase.f16_AerodynamicData.data.Cn.Cnr  ExtrapMethod=Clip  InternalRulePriority=Speed  RndMeth=Simplest
  CnrLefAlpha : Lookup_n-D  NumberOfTableDimensions=1  BreakpointsForDimension1=dataBase.f16_AerodynamicData.BP.Cn.deltaCnrlef.alpha  Table=dataBase.f16_AerodynamicData.data.Cn.deltaCnrlef  ExtrapMethod=Clip  InternalRulePriority=Speed  RndMeth=Simplest
  Constant : Constant  Value=0
  Constant1 : Constant  Value=2
  Constant{2..3,5..6} (4 alike) : Constant
  Constant4 : Constant  Value=2
  Divide : Product  Inputs=*/
  Divide1 : Product  Inputs=*/
  Divide2 : Product  Inputs=*/
  Gain : Gain  Gain=1/25
  Gain2 : Gain  Gain=1/20
  Gain3 : Gain  Gain=1/30
  MAC : Constant  Value=dataBase.MAC
  Product{,1..12} (13 alike) : Product
  Product13 : Product  Inputs=3
  Sum{,1..2,4..6,10..11} (8 alike) : Sum  Inputs=|+-
  Sum3 : Sum  Inputs=|+--
  Sum7 : Sum  Inputs=|++
  Sum8 : Sum  Inputs=|++
  Sum9 : Sum  Inputs=|++
  Wing Span : Constant  Value=dataBase.b
  Wing Span1 : Constant  Value=dataBase.b
  b : Constant  Value=dataBase.b
  Cn : Outport
  wires:
  States/1 -> Bus Selector/1
  [Velocity] -> Product2/2
  Product2/1 -> Divide/2
  [R] -> Product/1
  Constant1/1 -> Product2/1
  Wing Span/1 -> Product/2
  Wing Span1/1 -> Product8/2
  [P] -> Product8/1
  Constant4/1 -> Product9/1
  Product8/1 -> Divide1/1
  Divide1/1 -> [DimensionlessRollRate]
  Product9/1 -> Divide1/2
  Divide/1 -> [DimensionlessYawRate]
  Product/1 -> Divide/1
  [Velocity] -> Product9/2
  [LeadingEdgeFlap] -> Gain/1
  Gain2/1 -> [AileronDeflectionDelta]
  [Aileron] -> Gain2/1
  [Rudder] -> Gain3/1
  Gain3/1 -> [RudderDeflectionDelta]
  Gain/1 -> [LeadingEdgeFlapDeflectionDelta]
  [HorizontalTail] -> Cn(alpha,beta,ht)/3
  [Alpha] -> Cn(alpha,beta,ht)/1
  [Beta] -> Cn(alpha,beta,ht)/2
  Cn(alpha,beta,ht)/1 -> [CnAlphaBetaHt]
  Cn(alpha,beta,ht=0)/1 -> [CnAlphaBetaHt0]
  [Beta] -> Cn(alpha,beta,ht=0)/2
  [Alpha] -> Cn(alpha,beta,ht=0)/1
  Constant/1 -> Cn(alpha,beta,ht=0)/3
  [Beta] -> CnLef/2
  CnLef/1 -> [CnLefAlphaBeta]
  [Alpha] -> CnLef/1
  [Alpha] -> Cnda20/1
  [Beta] -> Cnda20/2
  Cnda20/1 -> [Cnda20AlphaBeta]
  Cndr30/1 -> [Cndr30AlphaBeta]
  [Beta] -> Cndr30/2
  [Alpha] -> Cndr30/1
  Cnda20Lef/1 -> [Cnda20LefAlphaBeta]
  [Beta] -> Cnda20Lef/2
  [Alpha] -> Cnda20Lef/1
  [CnLefAlphaBeta] -> Sum/1
  [CnAlphaBetaHt0] -> Sum/2
  Sum/1 -> [deltaCnLef]
  Sum1/1 -> [deltaCnda20]
  [CnAlphaBetaHt0] -> Sum1/2
  [Cnda20AlphaBeta] -> Sum1/1
  [Cndr30AlphaBeta] -> Sum2/1
  [CnAlphaBetaHt0] -> Sum2/2
  Sum2/1 -> [deltaCndr30]
  [Cnda20LefAlphaBeta] -> Sum3/1
  [CnLefAlphaBeta] -> Sum3/2
  [deltaCnda20] -> Sum3/3
  Sum3/1 -> [deltaCnda20Lef]
  Product5/1 -> Add1/4
  Add1/1 -> Cn/1
  [LeadingEdgeFlapDeflectionDelta] -> Sum10/2
  [LeadingEdgeFlapDeflectionDelta] -> Sum5/2
  Sum10/1 -> Product6/2
  [deltaCnLef] -> Product5/1
  [LeadingEdgeFlapDeflectionDelta] -> Sum6/2
  Constant6/1 -> Sum10/1
  Constant5/1 -> Sum6/1
  Product1/1 -> Sum9/2
  [CnpAlpha] -> Sum8/1
  Product6/1 -> Sum8/2
  Sum5/1 -> Product5/2
  [deltaCnrLefAlpha] -> Product10/1
  Product4/1 -> Add1/3
  Constant2/1 -> Sum4/1
  [deltaCnpLefAlpha] -> Product6/1
  Sum4/1 -> Product1/2
  [LeadingEdgeFlapDeflectionDelta] -> Sum4/2
  Product7/1 -> Add1/6
  [DimensionlessYawRate] -> Product11/2
  Constant3/1 -> Sum5/1
  [DimensionlessRollRate] -> Product7/2
  Sum7/1 -> Product11/1
  Sum8/1 -> Product7/1
  Product11/1 -> Add1/5
  [CnrAlpha] -> Sum7/1
  [deltaCndr30] -> Product4/1
  Product10/1 -> Sum7/2
  Sum9/1 -> Product3/1
  Product3/1 -> Add1/2
  [deltaCnda20] -> Sum9/1
  Sum6/1 -> Product10/2
  [RudderDeflectionDelta] -> Product4/2
  [deltaCnda20Lef] -> Product1/1
  [CnAlphaBetaHt] -> Add1/1
  [AileronDeflectionDelta] -> Product3/2
  CnrAlpha/1 -> [CnrAlpha]
  [Alpha] -> CnrAlpha/1
  [Alpha] -> CnpAlpha/1
  CnpAlpha/1 -> [CnpAlpha]
  CnpLefAlpha/1 -> [deltaCnpLefAlpha]
  [Alpha] -> CnpLefAlpha/1
  [Alpha] -> CnrLefAlpha/1
  CnrLefAlpha/1 -> [deltaCnrLefAlpha]
  [Alpha] -> CnBetaAlpha/1
  CnBetaAlpha/1 -> [deltaCnBetaAlpha]
  [deltaCnBetaAlpha] -> Product12/1
  [Beta] -> Product12/2
  Product12/1 -> Add1/7
  CGref/1 -> Sum11/1
  Sum11/1 -> Product13/2
  CG/1 -> Sum11/2
  b/1 -> Divide2/2
  MAC/1 -> Divide2/1
  Divide2/1 -> Product13/3
  [CY] -> Product13/1
  Product13/1 -> Add1/8
  Bus Selector/1 -> [Alpha]  "<Alpha>"
  Bus Selector/2 -> [Beta]  "<Beta>"
  Bus Selector/4 -> [R]  "<R>"
  Bus Selector/3 -> [P]  "<P>"
  Bus Selector/5 -> [HorizontalTail]  "<Horizontal Tail>"
  Bus Selector/6 -> [Aileron]  "<Aileron>"
  Bus Selector/7 -> [Rudder]  "<Rudder>"
  Bus Selector/8 -> [LeadingEdgeFlap]  "<LEF>"
  Bus Selector/9 -> [Velocity]  "<Velocity>"
  Bus Selector/10 -> [CY]  "<CY>"

== system F16_Quaternion/Equations of Motion (Quat)/Acisal_Ivme_Hesaplari/Subsystem ==
  p q r : Inport
  Inertia : Inport  Port=2
  Product : Product  Multiplication=Matrix(*)  InputSameDT=on  SaturateOnIntegerOverflow=on  OutDataTypeStr=Inherit: Same as first input
  Reshape1 : Reshape  OutputDimensionality=Column vector (2-D)
  Reshape2 : Reshape
  I * w : Outport  VectorParamsAs1DForOutWhenUnconnected=off
  wires:
  Inertia/1 -> Product/1
  p q r/1 -> Reshape1/1
  Reshape2/1 -> I * w/1
  Reshape1/1 -> Product/2
  Product/1 -> Reshape2/1

== matlab function F16_Quaternion/Atmosphere Model/MATLAB Function ==
  data: h input; g output; V input; T output; P output; rho output; Qdyn output; M output; speedOfSound output
%% Atmospheric Model

function [g,T,P,rho,Qdyn,M,speedOfSound] = fcn(h,V)

g = 9.80665*(6371020/(6371020+h))^2;
T = 288.15 - 6.5*h/1000;
P = 101325*(T/288.15)^(g/1.86584);
rho = P/(287.053*T);
k = 1.4;
R_c = 287.06;
speedOfSound = sqrt(k*R_c*T);
M = V/speedOfSound;
Qdyn = 0.5*rho*V^2;

== matlab function F16_Quaternion/Mass & Inertia/MATLAB Function ==
  data: Mass output; inertiaTensor output
function [Mass,inertiaTensor] = fcn()

%% Mass
Mass = 91188/9.8065; % kg

%% Moments of Inertia
Ixx = 12875; % kgm^2
Iyy = 75674; % kgm^2
Izz = 85552; % kgm^2
Ixz = 1331; % kgm^2
Ixy = 0; % kgm^2
Iyz = 0; % kgm^2

Izx = Ixz*(-1);
Iyx = Ixy*(-1);
Izy = Iyz*(-1);

%% Inertia Tensor
inertiaTensor = [Ixx, Ixy, Ixz;
                 Iyx, Iyy, Iyz;
                 Izx, Izy, Izz];

== matlab function F16_Quaternion/Propulsion Model/MATLAB Function ==
  data: Q input; T_moment output; R input




function T_moment = fcn(Q,R)

He = 216.9;

T_moment = [0 ; -He*R; He*Q];

== matlab function F16_Quaternion/Propulsion Model/MATLAB Function1 ==
  data: Tidle input size=1; Thrust output size=1; Tmil input size=1; Tmax input size=1; Throttle input size=1
function Thrust = fcn(Tidle, Tmil, Tmax, Throttle)

if Throttle <= 77
    Pc = 64.94*Throttle/100;
elseif Throttle > 77
    Pc = 217.38*Throttle/100 - 117.38;
else
    Pc = 0;
end

if Pc < 50
    Thrust = Tidle + (Tmil - Tidle)*Pc/50;
elseif 50 <= Pc
    Thrust = Tmil + (Tmax - Tmil)*(Pc-50)/50;
else
    Thrust = 0;
end
